simulink model "exampleKinematicViscosity"  (Simulink 7.6)
settings: Solver=ode45  StartTime=0.0  StopTime=10.0  RelTol=1e-3
libraries: carnot x4
settings Model: Creator=drhf  LastModifiedBy=drhf

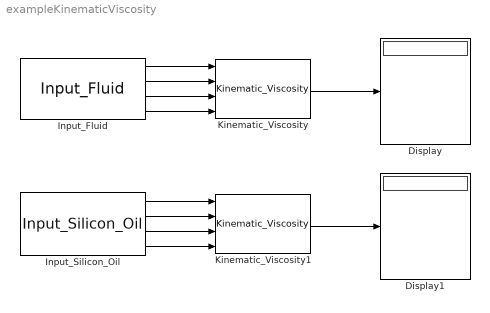
== system exampleKinematicViscosity ==
  Display : Display
  Display1 : Display
  Input_Fluid : carnot/Basic/Material_Properties/Input_Fluid  SystemSampleTime=-1  fluid=water  T=[10:10:50]  p=1e5  x=0.005
  Input_Silicon_Oil : carnot/Basic/Material_Properties/Input_Silicon_Oil  SystemSampleTime=-1  T=[10:10:50]  p=1e5
  Kinematic_Viscosity : carnot/Basic/Material_Properties/Kinematic_Viscosity  SystemSampleTime=-1
  Kinematic_Viscosity1 : carnot/Basic/Material_Properties/Kinematic_Viscosity  SystemSampleTime=-1
  wires:
  Input_Fluid/1 -> Kinematic_Viscosity/1
  Input_Fluid/2 -> Kinematic_Viscosity/2
  Input_Fluid/3 -> Kinematic_Viscosity/3
  Input_Fluid/4 -> Kinematic_Viscosity/4
  Kinematic_Viscosity/1 -> Display/1
  Input_Silicon_Oil/1 -> Kinematic_Viscosity1/1
  Input_Silicon_Oil/2 -> Kinematic_Viscosity1/2
  Input_Silicon_Oil/3 -> Kinematic_Viscosity1/3
  Input_Silicon_Oil/4 -> Kinematic_Viscosity1/4
  Kinematic_Viscosity1/1 -> Display1/1
